simulink model "single_thruster"  (R2023a)
settings: Solver=VariableStepAuto  StartTime=0.0  StopTime=40  RelTol=1e-3
undefined symbols (not defined in the file or in its folder): MarineRoboticsLib, T200, t200_force_n, t200_pwm_n
libraries: simulink x1
settings Model: Creator=dnad  LastModifiedBy=Pero
settings OptimizationCC: ReuseModelBlockBuffer=off

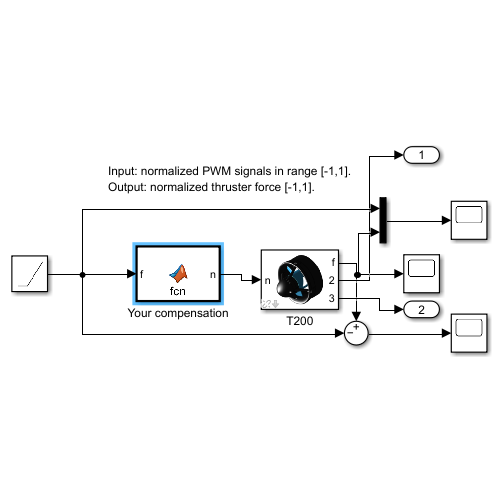
[thumbnail: Simulink's stored preview of the top-level diagram]
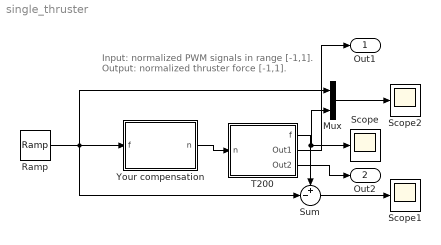
== system single_thruster ==
  note: Input: normalized PWM signals in range [-1,1].
      | Output: normalized thruster force [-1,1].
  Mux : Mux  Inputs=2
  Ramp : simulink/Sources/Ramp  slope=0.1  start=1  InitialOutput=-0.7
  Scope : Scope
  Scope1 : Scope
  Scope2 : Scope
  Sum : Sum  Inputs=+-|
  T200 : Subsystem  AncestorBlock=MarineRoboticsLib/T200  mask(T200){Keff=1, Tm=0}
      mask prompts: Keff "Efficiency"; Tm "ESC time constant (Tm)"
      mask help: This simulink block simulates a Blue Robotics T200 thruster on 14V controlled input. The efficiancy parameter given from [0,1] additionally decreases the force output of the thruster. The ESC reaction time is the time constant of the PT1 element included in the model. Put the time constant to zero to have instantaneous response.
      settings: LibrarySourceBlock=MarineRoboticsLib/T200
      mask Display: image('$imagefile'); % Use "Edit Image" on toolstrip to change.
  Your compensation : MATLAB Function  TreatAsAtomicUnit=on
  Out1 : Outport
  Out2 : Outport  Port=2
  wires:
  Ramp/1 -> Your compensation/1(f), Sum/2, Mux/1
  Mux/1 -> Scope2/1
  Sum/1 -> Scope1/1
  Your compensation/1(n) -> T200/1(n)
  T200/1(f) -> Mux/2, Scope/1, Sum/1
  T200/2(Out1) -> Out1/1
  T200/3(Out2) -> Out2/1

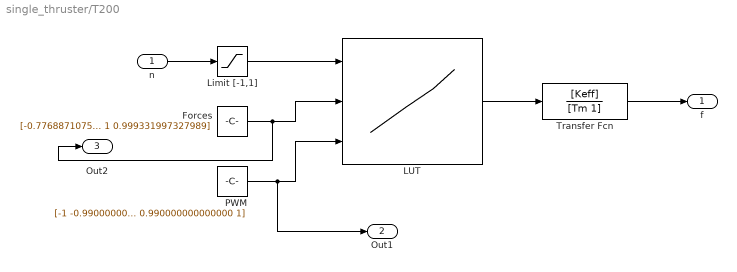
== system single_thruster/T200 ==
  n : Inport
  Forces : Constant  Value=|
      | [-0.776887107548430
      | -0.772545090180361
      | -0.771543086172345
      | -0.762525050100200
      | -0.751503006012024
      | -0.741482965931864
      | -0.727454909819639
      | -0.717434869739479
      | -0.704408817635270
      | -0.693386773547094
      | -0.684368737474950
      | -0.675350701402806
      | -0.663326653306613
      | -0.649298597194389
      | -0.637274549098196
      | -0.629258517034068
      | -0.614228456913828
      | -0.610220440881764
      | -0.594188376753507
      | -0.584168336673347
      | -0.573146292585170
      | -0.558116232464930
      | -0.550100200400802
      | -0.542084168336673
      | -0.532064128256513
      | -0.519038076152305
      | -0.516032064128256
      | -0.498997995991984
      | -0.486973947895792
      | -0.480961923847695
      | -0.467935871743487
      | -0.453907815631262
      | -0.447895791583166
      | -0.438877755511022
      | -0.421843687374750
      | -0.417835671342685
      | -0.401803607214429
      | -0.389779559118237
      | -0.379759519038076
      | -0.371743486973948
      | -0.360721442885772
      | -0.348697394789579
      | -0.345691382765531
      | -0.335671342685371
      | -0.326653306613226
      | -0.318637274549098
      | -0.309619238476954
      | -0.302605210420842
      | -0.292585170340681
      | -0.283567134268537
      | -0.273547094188377
      | -0.263527054108217
      | -0.257515030060120
      | -0.248496993987976
      | -0.240480961923848
      | -0.232464929859719
      | -0.224448897795591
      | -0.217434869739479
      | -0.210420841683367
      | -0.202404809619238
      | -0.195390781563126
      | -0.187374749498998
      | -0.178356713426854
      | -0.169338677354709
      | -0.163326653306613
      | -0.155310621242485
      | -0.150300601202405
      | -0.143286573146293
      | -0.137274549098196
      | -0.129258517034068
      | -0.121242484969940
      | -0.114228456913828
      | -0.108216432865731
      | -0.102204408817635
      | -0.0941883767535070
      | -0.0881763527054108
      | -0.0821643286573146
      | -0.0771543086172345
      | -0.0701402805611222
      | -0.0631262525050100
      | -0.0571142284569138
      | -0.0521042084168337
      | -0.0460921843687375
      | -0.0410821643286573
      | -0.0360721442885772
      | -0.0320641282565130
      | -0.0270541082164329
      | -0.0220440881763527
      | -0.0180360721442886
      | -0.0150300601202405
      | -0.0100200400801603
      | -0.00701402805611223
      | 0
      | 0
      | 0
      | 0
      | 0
      | 0
      | 0
      | 0
      | 0
      | 0
      | 0
      | 0
      | 0
      | 0
      | 0
      | 0
      | 0
      | 0.0100200400801603
      | 0.0140280561122245
      | 0.0180360721442886
      | 0.0220440881763527
      | 0.0270541082164329
      | 0.0320641282565130
      | 0.0390781563126253
      | 0.0440881763527054
      | 0.0501002004008016
      | 0.0581162324649299
      | 0.0641282565130261
      | 0.0721442885771543
      | 0.0801603206412826
      | 0.0871743486973948
      | 0.0941883767535070
      | 0.102204408817635
      | 0.110220440881764
      | 0.117234468937876
      | 0.127254509018036
      | 0.137274549098196
      | 0.142284569138277
      | 0.152304609218437
      | 0.160320641282565
      | 0.169338677354709
      | 0.182364729458918
      | 0.187374749498998
      | 0.196392785571142
      | 0.203406813627254
      | 0.213426853707415
      | 0.220440881763527
      | 0.232464929859719
      | 0.241482965931864
      | 0.252505010020040
      | 0.265531062124249
      | 0.272545090180361
      | 0.282565130260521
      | 0.292585170340681
      | 0.301603206412826
      | 0.310621242484970
      | 0.322645290581162
      | 0.333667334669339
      | 0.342685370741483
      | 0.354709418837675
      | 0.364729458917836
      | 0.377755511022044
      | 0.388777555110220
      | 0.400801603206413
      | 0.408817635270541
      | 0.421843687374750
      | 0.433867735470942
      | 0.442885771543086
      | 0.460921843687375
      | 0.467935871743487
      | 0.476953907815631
      | 0.495991983967936
      | 0.501002004008016
      | 0.517034068136273
      | 0.536072144288577
      | 0.553106212424850
      | 0.566132264529058
      | 0.582164328657315
      | 0.587174348697395
      | 0.609218436873748
      | 0.614228456913828
      | 0.636272545090180
      | 0.648296593186373
      | 0.661322645290581
      | 0.673346693386774
      | 0.691382765531062
      | 0.704408817635271
      | 0.714428857715431
      | 0.734468937875751
      | 0.742484969939880
      | 0.755511022044088
      | 0.771543086172345
      | 0.787575150300601
      | 0.800601202404810
      | 0.814629258517034
      | 0.832665330661323
      | 0.847695390781563
      | 0.866733466933868
      | 0.879759519038076
      | 0.889779559118237
      | 0.907815631262525
      | 0.917835671342685
      | 0.930861723446894
      | 0.950901803607214
      | 0.967935871743487
      | 0.976953907815631
      | 0.995991983967936
      | 1
      | 0.999331997327989]
  LUT : Lookup_n-D  NumberOfTableDimensions=1  BreakpointsForDimension1Source=Input port  BreakpointsForDimension1=t200_pwm_n  TableSource=Input port  Table=t200_force_n  InternalRulePriority=Speed  RndMeth=Simplest
      settings: InputPortMap=u0,p221,p5
  Limit [-1,1] : Saturate  UpperLimit=1  LowerLimit=-1
  PWM : Constant  Value=|
      | [-1
      | -0.990000000000000
      | -0.980000000000000
      | -0.970000000000000
      | -0.960000000000000
      | -0.950000000000000
      | -0.940000000000000
      | -0.930000000000000
      | -0.920000000000000
      | -0.910000000000000
      | -0.900000000000000
      | -0.890000000000000
      | -0.880000000000000
      | -0.870000000000000
      | -0.860000000000000
      | -0.850000000000000
      | -0.840000000000000
      | -0.830000000000000
      | -0.820000000000000
      | -0.810000000000000
      | -0.800000000000000
      | -0.790000000000000
      | -0.780000000000000
      | -0.770000000000000
      | -0.760000000000000
      | -0.750000000000000
      | -0.740000000000000
      | -0.730000000000000
      | -0.720000000000000
      | -0.710000000000000
      | -0.700000000000000
      | -0.690000000000000
      | -0.680000000000000
      | -0.670000000000000
      | -0.660000000000000
      | -0.650000000000000
      | -0.640000000000000
      | -0.630000000000000
      | -0.620000000000000
      | -0.610000000000000
      | -0.600000000000000
      | -0.590000000000000
      | -0.580000000000000
      | -0.570000000000000
      | -0.560000000000000
      | -0.550000000000000
      | -0.540000000000000
      | -0.530000000000000
      | -0.520000000000000
      | -0.510000000000000
      | -0.500000000000000
      | -0.490000000000000
      | -0.480000000000000
      | -0.470000000000000
      | -0.460000000000000
      | -0.450000000000000
      | -0.440000000000000
      | -0.430000000000000
      | -0.420000000000000
      | -0.410000000000000
      | -0.400000000000000
      | -0.390000000000000
      | -0.380000000000000
      | -0.370000000000000
      | -0.360000000000000
      | -0.350000000000000
      | -0.340000000000000
      | -0.330000000000000
      | -0.320000000000000
      | -0.310000000000000
      | -0.300000000000000
      | -0.290000000000000
      | -0.280000000000000
      | -0.270000000000000
      | -0.260000000000000
      | -0.250000000000000
      | -0.240000000000000
      | -0.230000000000000
      | -0.220000000000000
      | -0.210000000000000
      | -0.200000000000000
      | -0.190000000000000
      | -0.180000000000000
      | -0.170000000000000
      | -0.160000000000000
      | -0.150000000000000
      | -0.140000000000000
      | -0.130000000000000
      | -0.120000000000000
      | -0.110000000000000
      | -0.100000000000000
      | -0.0900000000000000
      | -0.0800000000000000
      | -0.0700000000000000
      | -0.0600000000000000
      | -0.0500000000000000
      | -0.0400000000000000
      | -0.0300000000000000
      | -0.0200000000000000
      | -0.0100000000000000
      | 0
      | 0.0100000000000000
      | 0.0200000000000000
      | 0.0300000000000000
      | 0.0400000000000000
      | 0.0500000000000000
      | 0.0600000000000000
      | 0.0700000000000000
      | 0.0800000000000000
      | 0.0900000000000000
      | 0.100000000000000
      | 0.110000000000000
      | 0.120000000000000
      | 0.130000000000000
      | 0.140000000000000
      | 0.150000000000000
      | 0.160000000000000
      | 0.170000000000000
      | 0.180000000000000
      | 0.190000000000000
      | 0.200000000000000
      | 0.210000000000000
      | 0.220000000000000
      | 0.230000000000000
      | 0.240000000000000
      | 0.250000000000000
      | 0.260000000000000
      | 0.270000000000000
      | 0.280000000000000
      | 0.290000000000000
      | 0.300000000000000
      | 0.310000000000000
      | 0.320000000000000
      | 0.330000000000000
      | 0.340000000000000
      | 0.350000000000000
      | 0.360000000000000
      | 0.370000000000000
      | 0.380000000000000
      | 0.390000000000000
      | 0.400000000000000
      | 0.410000000000000
      | 0.420000000000000
      | 0.430000000000000
      | 0.440000000000000
      | 0.450000000000000
      | 0.460000000000000
      | 0.470000000000000
      | 0.480000000000000
      | 0.490000000000000
      | 0.500000000000000
      | 0.510000000000000
      | 0.520000000000000
      | 0.530000000000000
      | 0.540000000000000
      | 0.550000000000000
      | 0.560000000000000
      | 0.570000000000000
      | 0.580000000000000
      | 0.590000000000000
      | 0.600000000000000
      | 0.610000000000000
      | 0.620000000000000
      | 0.630000000000000
      | 0.640000000000000
      | 0.650000000000000
      | 0.660000000000000
      | 0.670000000000000
      | 0.680000000000000
      | 0.690000000000000
      | 0.700000000000000
      | 0.710000000000000
      | 0.720000000000000
      | 0.730000000000000
      | 0.740000000000000
      | 0.750000000000000
      | 0.760000000000000
      | 0.770000000000000
      | 0.780000000000000
      | 0.790000000000000
      | 0.800000000000000
      | 0.810000000000000
      | 0.820000000000000
      | 0.830000000000000
      | 0.840000000000000
      | 0.850000000000000
      | 0.860000000000000
      | 0.870000000000000
      | 0.880000000000000
      | 0.890000000000000
      | 0.900000000000000
      | 0.910000000000000
      | 0.920000000000000
      | 0.930000000000000
      | 0.940000000000000
      | 0.950000000000000
      | 0.960000000000000
      | 0.970000000000000
      | 0.980000000000000
      | 0.990000000000000
      | 1]
  Transfer Fcn : TransferFcn  Numerator=[Keff]  Denominator=[Tm 1]
  f : Outport
  Out1 : Outport  Port=2
  Out2 : Outport  Port=3
  wires:
  PWM/1 -> Out1/1, LUT/3
  Forces/1 -> Out2/1, LUT/2
  Transfer Fcn/1 -> f/1
  n/1 -> Limit [-1,1]/1
  LUT/1 -> Transfer Fcn/1
  Limit [-1,1]/1 -> LUT/1

== matlab function single_thruster/Your compensation ==
  data: f input; n output
function n = fcn(f)

%p1 = -0.0262;
%p2 = 0.4569;
%p3 = 0.1381;
%p4 = 0.4963;
%p5 = 0.0014;

p1 = 0.5869;
p2 = -0.9109;
p3 = -0.3809;
p4 = 1.6743;
p5 = -0.0089;

n = p1*f^4 + p2*f^3 + p3*f^2 + p4*f + p5;
%n = f;

end
